simulink model "MPPT"  (R2021a)
settings: Solver=VariableStepAuto  StartTime=0.0  StopTime=250  RelTol=1e-3
libraries: spsSeriesRLCBranchLib x4, spsCurrentMeasurementLib x1, spsDiodeLib x1, spsIGBTDiodeLib x1, spsPVArrayLib x1, spsPWMGeneratorDCDCLib x1, spsVoltageMeasurementLib x1, simulink x1, spspowerguiLib x1
settings Model: Creator=suraj kumar  LastModifiedBy=suraj kumar

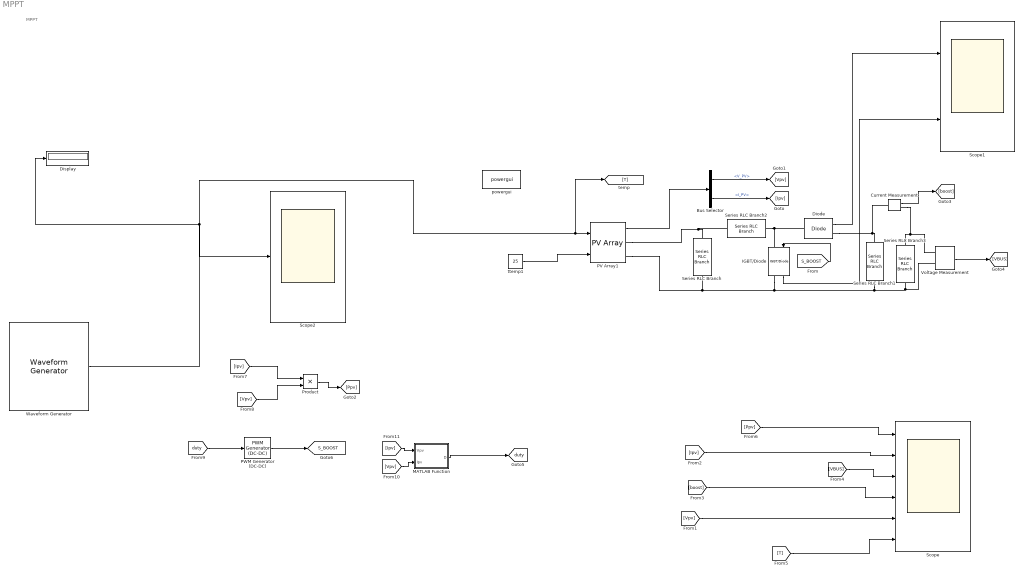
== system MPPT ==
  note: MPPT
  Bus Selector : BusSelector  OutputSignals=V_PV,I_PV
  Current Measurement : spsCurrentMeasurementLib/Current Measurement  PhasorSimulation=off  OutputType=Complex  PSBequivalent=0
  Diode : spsDiodeLib/Diode  Ron=0.001  Lon=0  Vf=0.8  IC=0  UseSnubber=0  Rs=500  Cs=250e-9  Measurements=on
  Display : Display
  IGBT/Diode : spsIGBTDiodeLib/IGBT//Diode  Ron=1e-3  Rs=1e5  Cs=inf  Measurements=on
  MATLAB Function : MATLAB Function  TreatAsAtomicUnit=on
  PV Array1 : spsPVArrayLib/PV Array  Npar=5  Nser=1  PlotType=array @ 1000 W/m2 & specified temperatures  S_vec="[ 1000  500  100 ]"  Temp_C_vec="[ 45 25  ]"  ModuleName=User-defined  PlotWhenSelected=off  Pm=213.15  Ncell=60  Voc=36.3  Isc=7.84  Vm=29  Im=7.35  beta_Voc_pc=-0.36099  alpha_Isc_pc=0.102  beta_Voc=-0.13104  alpha_Isc=0.0079968  IL=7.8654  I0=2.9273e-10  nI=0.98119  Rsh=313.0553  Rs=0.39381  RobustModel=off  RobustCellTemperature=25  BAL=on  Tc=1e-6  Tfilter=5e-5
  PWM Generator (DC-DC) : spsPWMGeneratorDCDCLib/PWM Generator (DC-DC)  Fsw=5000  Ts=10e-5
  Product : Product
  Scope : Scope  NumInputPorts=6
  Scope1 : Scope  NumInputPorts=2
  Scope2 : Scope
  Series RLC Branch : spsSeriesRLCBranchLib/Series RLC Branch  LConnTagsString=__new0  RConnTagsString=__new0  BranchType=RC  Resistance=1e-4  Inductance=1e-3  SetiL0=off  InitialCurrent=0  Capacitance=1000e-5  Setx0=off  InitialVoltage=0  Measurements=None
  Series RLC Branch1 : spsSeriesRLCBranchLib/Series RLC Branch  LConnTagsString=__new0  RConnTagsString=__new0  BranchType=RC  Resistance=1e-4  Inductance=1e-3  SetiL0=off  InitialCurrent=0  Capacitance=3300e-5  Setx0=off  InitialVoltage=0  Measurements=None
  Series RLC Branch2 : spsSeriesRLCBranchLib/Series RLC Branch  LConnTagsString=__new0  RConnTagsString=__new0  BranchType=RL  Resistance=0.1  Inductance=5e-3  SetiL0=off  InitialCurrent=0  Capacitance=1e-6  Setx0=off  InitialVoltage=0  Measurements=None
  Series RLC Branch3 : spsSeriesRLCBranchLib/Series RLC Branch  LConnTagsString=__new0  RConnTagsString=__new0  BranchType=R  Resistance=10  Inductance=1e-3  SetiL0=off  InitialCurrent=0  Capacitance=1e-6  Setx0=off  InitialVoltage=0  Measurements=None
  Voltage Measurement : spsVoltageMeasurementLib/Voltage Measurement  PhasorSimulation=off  OutputType=Complex  PSBequivalent=0
  Waveform Generator : simulink/Sources/Waveform Generator  OutMin=[]  OutMax=[]  OutDataTypeStr=double  SelectedSignal=1  Signals=sin(1000,0.262,0)#1000  BlockNames=MultiportSwitch_9dfe9e6dcfc2430#MultiportSwitch_12632df6e1b6439  SampleTime=0.1
  powergui : spspowerguiLib/powergui  Priority=1  SimulationMode=Discrete  SampleTime=10e-5  frequency=60  Iterations=50  frequencyindice=0  Pbase=100e6  ErrMax=1e-4  UnitsV=kV  UnitsW=MW  buscounter=0  FunctionMessages=off  echomessages=off  EnableUseOfTLC=off  CurrentSourceSwitches=off  DisableSnubberDevices=off  DisableRonSwitches=off  DisableVfSwitches=off  DisplayEquations=off  AutomaticDiscreteSolvers=off  SolverType=Tustin/Backward Euler (TBE)  Interpol=off  ExternalGateDelay=off  methode=off  Ts=100  x0status=blocks  SPID=on  SwTol=0  HookPort=off  NonlinearTolerance=1e-4  nMaxIteration=100  ContinueOnMaxIteration=off  RestoreLinks=warning  ResistiveCurrentMeasurement=off  Frange=[0:2:500]  Ylog=off  Xlog=on  ShowGrid=off  save=off  variable=ZData  structure=0  ZoomFFT=off  StartTime=0.0  cycles=1  DisplayStyle=1  fundamental=60  FreqAxis=off  MaxFrequency=1000  frequencyindicesteady=1  RmsSteady=1  display=off
  ttemp1 : Constant  Value=25
  tag scope: S_BOOST=global, duty=global
  wires:
  ttemp1/1 -> PV Array1/2
  PV Array1/1 -> Bus Selector/1
  Bus Selector/1 -> [Vpv]  "<V_PV>"
  Bus Selector/2 -> [Ipv]  "<I_PV>"
  Waveform Generator/1 -> [T], PV Array1/1, Display/1, Scope2/1
  Current Measurement/1 -> [boost]
  Voltage Measurement/1 -> [VBUS]
  [S_BOOST] -> IGBT/Diode/1
  [Vpv] -> Scope/5
  [Ipv] -> Scope/2
  [boost] -> Scope/4
  [VBUS] -> Scope/3
  [T] -> Scope/6
  [Ppv] -> Scope/1
  Product/1 -> [Ppv]
  [Ipv] -> Product/1
  [Vpv] -> Product/2
  PWM Generator (DC-DC)/1 -> [S_BOOST]
  [duty] -> PWM Generator (DC-DC)/1
  [Vpv] -> MATLAB Function/2(Ipv)
  [Ipv] -> MATLAB Function/1(Vpv)
  MATLAB Function/1(D) -> [duty]
  IGBT/Diode/1 -> Scope1/2
  Diode/1 -> Scope1/1
  connections:
  PV Array1/RConn1 -- Series RLC Branch2/RConn1 -- Series RLC Branch/LConn1
  PV Array1/RConn2 -- Voltage Measurement/LConn2 -- Series RLC Branch3/RConn1 -- Series RLC Branch1/RConn1 -- IGBT/Diode/RConn1 -- Series RLC Branch/RConn1
  Series RLC Branch2/LConn1 -- Diode/LConn1 -- IGBT/Diode/LConn1
  Diode/RConn1 -- Current Measurement/LConn1 -- Series RLC Branch1/LConn1
  Series RLC Branch3/LConn1 -- Current Measurement/RConn1 -- Voltage Measurement/LConn1

== matlab function MPPT/MATLAB Function ==
  data: Vpv input; Ipv input; D output
function D = pandO(Vpv,Ipv)

persistent Dprev Pprev Vprev

if isempty(Dprev)
    Dprev=0.7;
    Vprev=190;
    Pprev=2000;
end

deltaD =125e-6;

%calculate measured array power
Ppv=Vpv*Ipv;
%increase or decrease duty cycle based on conditions
if(Ppv-Pprev)~=0
    if(Ppv-Pprev)>0
        if(Vpv-Vprev)>0
            D=Dprev-deltaD;
        else
            D=Dprev+deltaD;
        end
    else
        if(Vpv-Vprev)>0
            D=Dprev+deltaD;
        else
            D=Dprev-deltaD;
        end
    end
    
else
    
    D=Dprev;
    
end
        %update internal values
        Dprev=D;
        Vprev=Vpv;
        Pprev=Ppv;
